simulink model "PI_Ctrl"  (R2020b)
settings: Solver=VariableStepAuto  StartTime=0.0  StopTime=10.0  RelTol=1e-3
PostLoadFcn:
  | a = -3;
  | b = -4;
  | Kp = 36;
  | Ki = 4;
  | m = 25;
  | t = [0:0.01:10]';
  | Ts = 0.01;
  | stin = [zeros(floor((length(t)/2)+1),1) ; 5*ones(floor(length(t)/2),1)];
  | itr = 200;
settings Model: Creator=vijay jagtap  LastModifiedBy=vijay jagtap

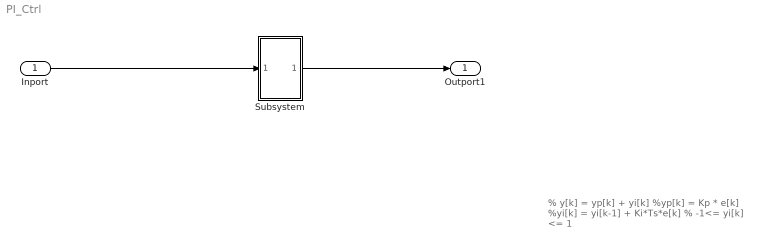
== system PI_Ctrl ==
  note: % y[k] = yp[k] + yi[k]
      | %yp[k] = Kp * e[k]
      | %yi[k] = yi[k-1] + Ki*Ts*e[k]
      | % -1<= yi[k] <= 1
  Inport : Inport  OutDataTypeStr=double  PortDimensions=1  SampleTime=0
  Subsystem : Subsystem  mask{Kp=25, Ki=300, Ts=0.01}
  Outport1 : Outport  OutDataTypeStr=double  PortDimensions=1  SampleTime=0
  wires:
  Inport/1 -> Subsystem/1(In1)
  Subsystem/1(y_k) -> Outport1/1

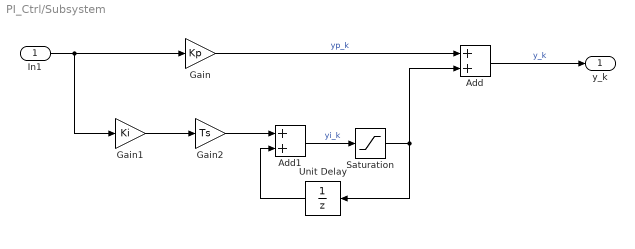
== system PI_Ctrl/Subsystem ==
  In1 : Inport
  Add : Sum
  Add1 : Sum
  Gain : Gain  Gain=Kp
  Gain1 : Gain  Gain=Ki
  Gain2 : Gain  Gain=Ts
  Saturation : Saturate  UpperLimit=1  LowerLimit=-1
  Unit Delay : UnitDelay  SampleTime=-1  HasFrameUpgradeWarning=on
  y_k : Outport
  wires:
  In1/1 -> Gain/1, Gain1/1
  Unit Delay/1 -> Add1/2
  Add1/1 -> Saturation/1  "yi_k"
  Add/1 -> y_k/1  "y_k"
  Gain2/1 -> Add1/1
  Gain/1 -> Add/1  "yp_k"
  Gain1/1 -> Gain2/1
  Saturation/1 -> Unit Delay/1, Add/2
